simulink model "rct_CSTR"  (R2022a)
settings: Solver=ode45  StartTime=0  StopTime=50  RelTol=1e-3  EnableMultiTasking=on
PreLoadFcn:
  | Ts = 0.5;
  | load CSTRData
model workspace (MAT data in the model file):
  Cr_vec = [2 2.5 3 3.5 4 4.5 5 5.5 6 6.5 7 7.5 8 8.5 9]
  Ki_vec = [-2 -2 -2 -2 -2 -2 -2 -2 -2 -2 -2 -2 -2 -2 -2]
  Kp_vec = [0 0 0 0 0 0 0 0 0 0 0 0 0 0 0]
  Kt_vec = [0 0 0 0 0 0 0 0 0 0 0 0 0 0 0]
  a_vec = [0 0 0 0 0 0 0 0 0 0 0 0 0 0 0]
  b_vec = [0 0 0 0 0 0 0 0 0 0 0 0 0 0 0]
values from neighbouring files (symbols this model uses):
  CrEQ = linspace(8.57,2,5)'    [Gain_Scheduled_Control_of_a_Chemical_Reactor.m]
  TcEQ = zeros(5,1)    [Gain_Scheduled_Control_of_a_Chemical_Reactor.m]
  TrEQ = zeros(5,1)    [Gain_Scheduled_Control_of_a_Chemical_Reactor.m]
undefined symbols (not defined in the file or in its folder): DiscIntNeverNeededParam, sigbuilder_block
settings Model: Creator=The MathWorks, Inc.  LastModifiedBy=The MathWorks, Inc.
settings SolverCC: AlgebraicLoopSolver=TrustRegion  MaxZcPerStep=1
settings DataIOCC: InitialState=[311.267; 8.5695]  LimitDataPoints=on  SaveFormat=Array  ReturnWorkspaceOutputs=off  SignalLoggingName=logsOut
settings OptimizationCC: BooleanDataType=off  DefaultParameterBehavior=Inlined  InlineInvariantSignals=on  BufferReuse=off  ExpressionDepthLimit=2147483647  InitFltsAndDblsToZero=on  LifeSpan=inf
settings DebuggingCC: SaveWithParameterizedLinksMsg=none  UnderspecifiedInitializationDetection=Classic  MergeDetectMultiDrivingBlocksExec=none  CheckExecutionContextPreStartOutputMsg=on  SignalResolutionControl=TryResolveAllWithWarning  MultiTaskDSMMsg=warning  MultiTaskCondExecSysMsg=none  UnconnectedInputMsg=warning  UnconnectedOutputMsg=warning  UnconnectedLineMsg=warning  AllowSymbolicDim=off  StateNameClashWarn=warning  SFUnexpectedBacktrackingDiag=warning  SFNoUnconditionalDefaultTransitionDiag=warning  SFExecutionAtInitializationDiag=none  SFMachineParentedDataDiag=warning  ArithmeticOperatorsInVariantConditions=warning
settings HardwareCC: ProdBitPerPointer=32  ProdBitPerSizeT=32  ProdBitPerPtrDiffT=32  ProdLargestAtomicFloat=None  ProdIntDivRoundTo=Undefined  ProdEndianess=Unspecified  ProdWordSize=32  ProdHWDeviceType=32-bit Generic  TargetUnknown=on
settings ModelReferenceCC: PropagateSignalLabelsOutOfModel=off
settings SFSimCC: SimUseLocalCustomCode=off  CustomCodeUndefinedFunction=UseInterfaceOnly
settings RTWCC: RTWUseLocalCustomCode=off  DLArmComputeVersion=19.05
settings CodeAppCC: StateflowObjectComments=on
settings GRTTargetCC: TargetFcnLib=ansi_tfl_tmw.mat  TargetLangStandard=C89/C90 (ANSI)  CombineOutputUpdateFcns=off  GRTInterface=on
settings ConfigComp: CovMetricSettings=dw  CovSaveCumulativeToWorkspaceVar=on  CovSaveSingleToWorkspaceVar=on  CovExternalEMLEnable=off  CovSFcnEnable=off

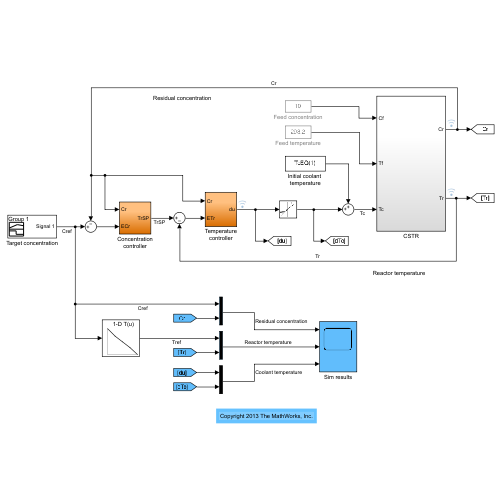
[thumbnail: Simulink's stored preview of the top-level diagram]
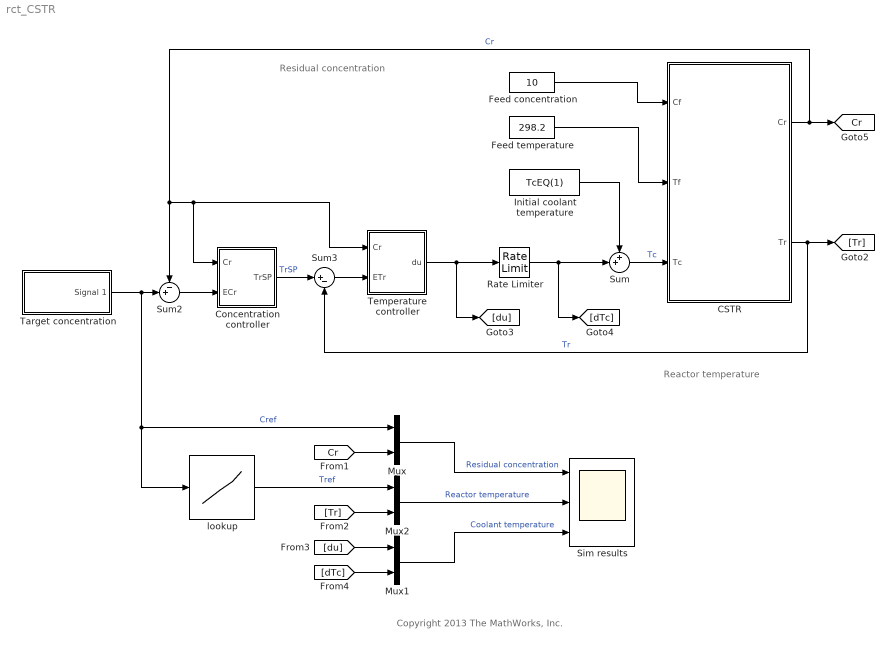
== system rct_CSTR ==
  note: Copyright 2013 The MathWorks, Inc.
  note: Reactor temperature
  note: Residual concentration
  CSTR : Subsystem
  Concentration controller : Subsystem
  Feed concentration : Constant  Value=10  SampleTime=0
  Feed temperature : Constant  Value=298.2  SampleTime=0
  Initial coolant temperature : Constant  Value=TcEQ(1)  SampleTime=0
  Mux : Mux  Inputs=2
  Mux1 : Mux  Inputs=2
  Mux2 : Mux  Inputs=2
  Rate Limiter : RateLimiter  RisingSlewLimit=10  FallingSlewLimit=-10  SampleTimeMode=inherited
  Sim results : Scope  NumInputPorts=3
  Sum : Sum  Inputs=++|
  Sum2 : Sum  Inputs=-+|
  Sum3 : Sum  Inputs=|+-
  Target concentration : Subsystem  Tag=STV Subsys  LoadFcn=sigbuilder_block('load');  StartFcn=sigbuilder_block('start');  StopFcn=sigbuilder_block('stop');  ClipboardFcn=sigbuilder_block('clipboard');  mask(Sigbuilder block){tuvar=[0:10]}
      mask help: Simulink:masks:SigbuilderBlock_MD
      mask init:
      | if ~strcmp(get_param(bdroot(gcbh),'SimulationStatus'),'stopped') tuvar = sigbuilder_block('maskInit'); end
      settings: CopyFcn=sigbuilder_block('copy');  DeleteFcn=sigbuilder_block('delete');  ModelCloseFcn=sigbuilder_block('modelClose');  PreSaveFcn=sigbuilder_block('preSave');  PauseFcn=sigbuilder_block('pause');  ContinueFcn=sigbuilder_block('continue');  NameChangeFcn=sigbuilder_block('namechange');  OpenFcn=sigbuilder_block('open',[358.5 207 550.5 395.25 ]);  CloseFcn=sigbuilder_block('close');
      mask Display: plot(0, 0, 100, 100,[2, 2, 32, 32, 2], [68, 8, 8, 68, 68],[32, 2], [38, 38], [32, 19, 2],[53, 60, 44], [32, 17, 17, 2],[16, 16, 31, 31]);txt = getActiveGroup(gcbh);text(2, 100, txt,'verticalAlignment', 'top');
  Temperature controller : Subsystem
  lookup : Lookup_n-D  NumberOfTableDimensions=1  LookupTableObject=''  BreakpointsForDimension1=flipud(CrEQ)  Table=flipud(TrEQ)  RndMeth=Simplest
  tag scope: Cr=global
  wires:
  Feed concentration/1 -> CSTR/1(Cf)
  Feed temperature/1 -> CSTR/2(Tf)
  CSTR/2(Tr) -> [Tr], Sum3/2  "Tr"
  Temperature controller/1(du) -> [du], Rate Limiter/1
  Mux1/1 -> Sim results/3  "Coolant temperature"
  Initial coolant temperature/1 -> Sum/1
  CSTR/1(Cr) -> [Cr], Temperature controller/1(Cr), Concentration controller/1(Cr), Sum2/1  "Cr"
  Target concentration/1(Signal 1) -> lookup/1, Mux/1, Sum2/2  "Cref"
  [Cr] -> Mux/2
  Mux2/1 -> Sim results/2  "Reactor temperature"
  Mux/1 -> Sim results/1  "Residual concentration"
  [du] -> Mux1/1
  [dTc] -> Mux1/2
  [Tr] -> Mux2/2
  Sum3/1 -> Temperature controller/2(ETr)
  lookup/1 -> Mux2/1  "Tref"
  Concentration controller/1(TrSP) -> Sum3/1  "TrSP"
  Sum/1 -> CSTR/3(Tc)  "Tc"
  Rate Limiter/1 -> Sum/2, [dTc]
  Sum2/1 -> Concentration controller/2(ECr)

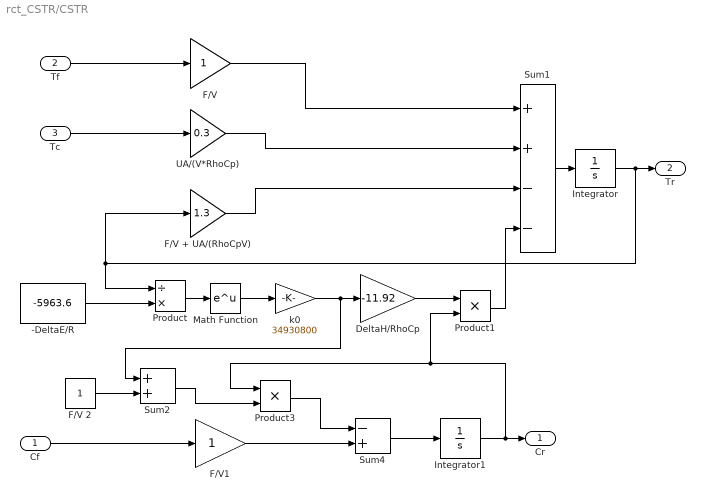
== system rct_CSTR/CSTR ==
  Cf : Inport
  Tf : Inport  Port=2
  Tc : Inport  Port=3
  -DeltaE/R : Constant  Value=-5963.6  SampleTime=0
  DeltaH/RhoCp : Gain  Gain=-11.92  SaturateOnIntegerOverflow=on  OutDataTypeStr=Inherit: Same as input  ParamDataTypeStr=Inherit: Same as input
  F/V : Gain  SaturateOnIntegerOverflow=on  OutDataTypeStr=Inherit: Same as input  ParamDataTypeStr=Inherit: Same as input
  F/V + UA/(RhoCpV) : Gain  Gain=1.3  SaturateOnIntegerOverflow=on  OutDataTypeStr=Inherit: Same as input  ParamDataTypeStr=Inherit: Same as input
  F/V 2 : Constant  SampleTime=0
  F/V1 : Gain  SaturateOnIntegerOverflow=on  OutDataTypeStr=Inherit: Same as input  ParamDataTypeStr=Inherit: Same as input
  Integrator : Integrator  InitialCondition=311.26  LimitOutput=on  LowerSaturationLimit=0
  Integrator1 : Integrator  InitialCondition=8.57  LimitOutput=on  LowerSaturationLimit=0
  Math Function : Math  SignedPower=on
  Product : Product  Inputs=/*  InputSameDT=on  RndMeth=Zero  SaturateOnIntegerOverflow=on  OutDataTypeStr=Inherit: Same as first input
  Product1 : Product  InputSameDT=on  RndMeth=Zero  SaturateOnIntegerOverflow=on  OutDataTypeStr=Inherit: Same as first input
  Product3 : Product  InputSameDT=on  RndMeth=Zero  SaturateOnIntegerOverflow=on  OutDataTypeStr=Inherit: Same as first input
  Sum1 : Sum  Inputs=++--  InputSameDT=on  SaturateOnIntegerOverflow=on  OutDataTypeStr=Inherit: Same as first input
  Sum2 : Sum  InputSameDT=on  SaturateOnIntegerOverflow=on  OutDataTypeStr=Inherit: Same as first input
  Sum4 : Sum  Inputs=-+  InputSameDT=on  SaturateOnIntegerOverflow=on  OutDataTypeStr=Inherit: Same as first input
  UA/(V*RhoCp) : Gain  Gain=0.3  SaturateOnIntegerOverflow=on  OutDataTypeStr=Inherit: Same as input  ParamDataTypeStr=Inherit: Same as input
  k0 : Gain  Gain=34930800  SaturateOnIntegerOverflow=on  OutDataTypeStr=Inherit: Same as input  ParamDataTypeStr=Inherit: Same as input
  Cr : Outport
  Tr : Outport  Port=2
  wires:
  F/V/1 -> Sum1/1
  Sum1/1 -> Integrator/1
  Integrator/1 -> Product/1, F/V + UA/(RhoCpV)/1, Tr/1
  UA/(V*RhoCp)/1 -> Sum1/2
  F/V + UA/(RhoCpV)/1 -> Sum1/3
  Product/1 -> Math Function/1
  Math Function/1 -> k0/1
  DeltaH/RhoCp/1 -> Product1/1
  Product1/1 -> Sum1/4
  k0/1 -> DeltaH/RhoCp/1, Sum2/1
  -DeltaE/R/1 -> Product/2
  Product3/1 -> Sum4/1
  Sum4/1 -> Integrator1/1
  Integrator1/1 -> Product1/2, Product3/1, Cr/1
  F/V 2/1 -> Sum2/2
  F/V1/1 -> Sum4/2
  Tf/1 -> F/V/1
  Cf/1 -> F/V1/1
  Tc/1 -> UA/(V*RhoCp)/1
  Sum2/1 -> Product3/2

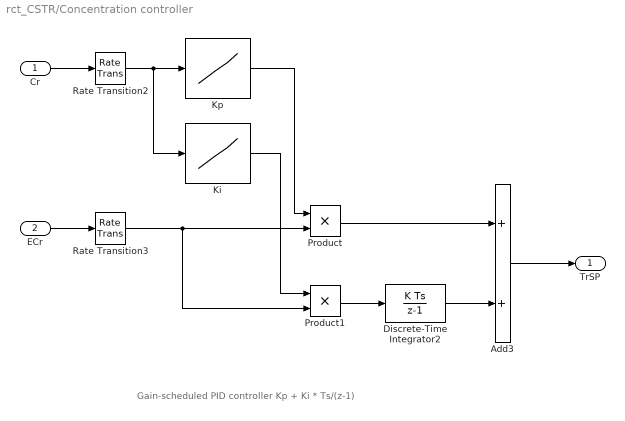
== system rct_CSTR/Concentration controller ==
  note: Gain-scheduled PID controller Kp + Ki * Ts/(z-1)
  Cr : Inport
  ECr : Inport  Port=2
  Add3 : Sum
  Discrete-Time Integrator2 : DiscreteIntegrator  InitialCondition=TrEQ(1)  SampleTime=Ts  ICPrevOutput=DiscIntNeverNeededParam  ICPrevScaledInput=DiscIntNeverNeededParam
  Ki : Lookup_n-D  NumberOfTableDimensions=1  LookupTableObject=''  BreakpointsForDimension1=Cr_vec  Table=Ki_vec  InternalRulePriority=Speed  RndMeth=Simplest
  Kp : Lookup_n-D  NumberOfTableDimensions=1  LookupTableObject=''  BreakpointsForDimension1=Cr_vec  Table=Kp_vec  InternalRulePriority=Speed  RndMeth=Simplest
  Product : Product
  Product1 : Product
  Rate Transition2 : RateTransition  OutPortSampleTime=Ts
  Rate Transition3 : RateTransition  OutPortSampleTime=Ts
  TrSP : Outport
  wires:
  ECr/1 -> Rate Transition3/1
  Discrete-Time Integrator2/1 -> Add3/2
  Product/1 -> Add3/1
  Add3/1 -> TrSP/1
  Cr/1 -> Rate Transition2/1
  Kp/1 -> Product/1
  Rate Transition2/1 -> Ki/1, Kp/1
  Product1/1 -> Discrete-Time Integrator2/1
  Rate Transition3/1 -> Product1/2, Product/2
  Ki/1 -> Product1/1

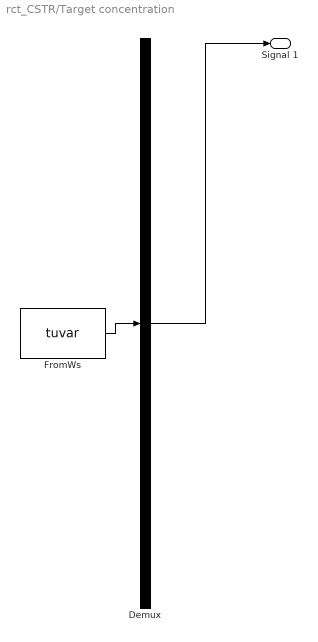
== system rct_CSTR/Target concentration ==
  Demux : Demux  Tag=STV Demux  Outputs=1
      settings: DisplayOption=none
  FromWs : FromWorkspace  Tag=STV FromWs  VariableName=tuvar
      SigBuilderData=|
      | common.afterFinalStr = 'Extrapolate'
      | common.sampleTime = 0
      | dataSet.timeRange = [0 45]
      | dataSet.name = 'Group 1'
      | sbobj.Groups.Name = 'Group 1'
      | sbobj.Groups.Signals.Name = 'Signal 1'
      | sbobj.Groups.Signals.XData = [0 10 36 45]
      | sbobj.Groups.Signals.YData = [8.57 8.57 2 2]
      | sbobj.Groups.TimeRange = [0 45]
  Signal 1 : Outport  Tag=STV Outport
  wires:
  Demux/1 -> Signal 1/1
  FromWs/1 -> Demux/1

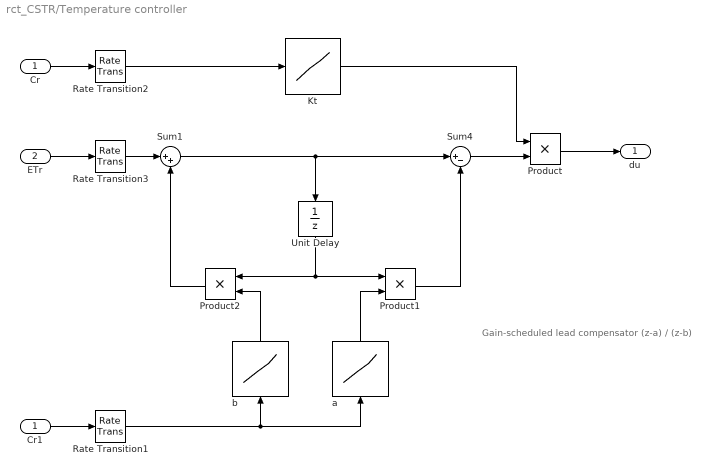
== system rct_CSTR/Temperature controller ==
  note: Gain-scheduled lead compensator
      | (z-a) / (z-b)
  Cr : Inport
  ETr : Inport  Port=2
  Cr1 : InportShadow
  Kt : Lookup_n-D  NumberOfTableDimensions=1  LookupTableObject=''  BreakpointsForDimension1=Cr_vec  Table=Kt_vec  InternalRulePriority=Speed  RndMeth=Simplest
  Product : Product
  Product1 : Product
  Product2 : Product
  Rate Transition1 : RateTransition  OutPortSampleTime=Ts
  Rate Transition2 : RateTransition  OutPortSampleTime=Ts
  Rate Transition3 : RateTransition  OutPortSampleTime=Ts
  Sum1 : Sum  Inputs=|++
  Sum4 : Sum  Inputs=|+-
  Unit Delay : UnitDelay  SampleTime=Ts  HasFrameUpgradeWarning=on
  a : Lookup_n-D  NumberOfTableDimensions=1  LookupTableObject=''  BreakpointsForDimension1=Cr_vec  Table=a_vec  InternalRulePriority=Speed  RndMeth=Simplest
  b : Lookup_n-D  NumberOfTableDimensions=1  LookupTableObject=''  BreakpointsForDimension1=Cr_vec  Table=b_vec  InternalRulePriority=Speed  RndMeth=Simplest
  du : Outport
  wires:
  Product/1 -> du/1
  Product1/1 -> Sum4/2
  Sum1/1 -> Sum4/1, Unit Delay/1
  Sum4/1 -> Product/2
  Product2/1 -> Sum1/2
  Unit Delay/1 -> Product1/1, Product2/1
  ETr/1 -> Rate Transition3/1
  Rate Transition3/1 -> Sum1/1
  Cr/1 -> Rate Transition2/1
  Rate Transition2/1 -> Kt/1
  Kt/1 -> Product/1
  Cr1/1 -> Rate Transition1/1
  a/1 -> Product1/2
  Rate Transition1/1 -> b/1, a/1
  b/1 -> Product2/2
